simulink model "Inverter2Motor"  (R2025a)
settings: Solver=VariableStepAuto  StartTime=0.0  StopTime=5  RelTol=1e-3
model workspace (MAT data in the model file):
  CT_AmpersPerLSB = 0.0515718
  InverterVdc = 440
  Max_ADC_CNT = 4096
  MotorBaseCurrent = 20
  MotorKe = 0.031
  MotorLd = 0.000247
  MotorLq = 0.000371
  MotorPoles = 4
  MotorRs = 0.126
  PI_params_idKi = 1000
  PI_params_idKp = 0.4
  PI_params_iqKi = 1000
  PI_params_iqKp = 0.6
  Ts = 5e-05
libraries: simulink x3, slpidlib x2, mcbplantlib x1, autolibpmsminterior x1, mcbcontrolslib x1, dspstat3 x1, mcbcontrollergainlib x1, spsRMSLib x1, mcbeeMathTransformLib x1
settings Model: Creator=taiji  LastModifiedBy=taiji
settings DebuggingCC: ParamSuppressDoubleToSinglePrecisionLossMsg=on
settings RTWCC: GenCodeOnly=on  Toolchain=MinGW64 | gmake (64-bit Windows)

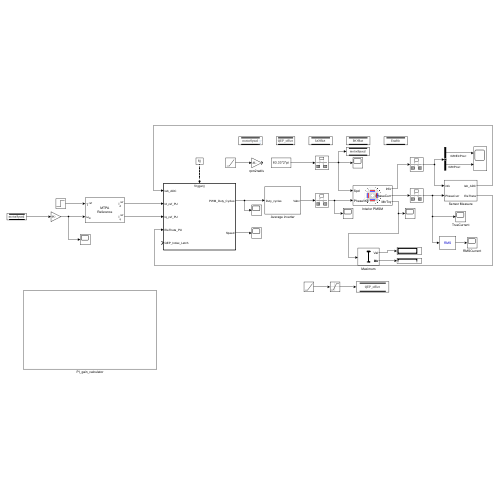
[thumbnail: Simulink's stored preview of the top-level diagram]
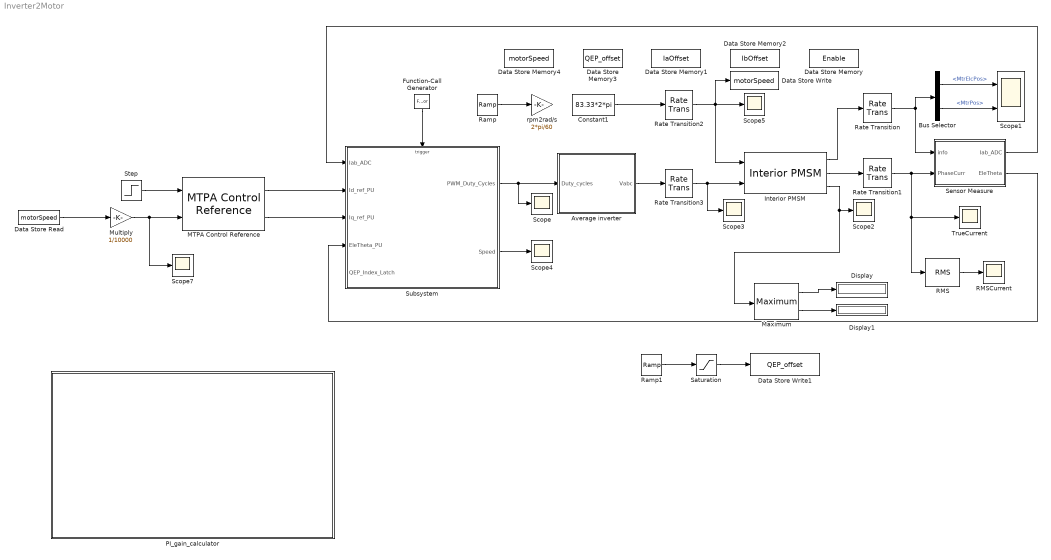
== system Inverter2Motor ==
  Average inverter : Subsystem
  Bus Selector : BusSelector  OutputSignals=MtrElcPos,MtrPos
  Constant1 : Constant  Value=83.33*2*pi
  Data Store Memory : DataStoreMemory  DataStoreName=Enable  WriteAfterWriteMsg=warning  InitialValue=1  ShowAdditionalParam=off  OutDataTypeStr=boolean
  Data Store Memory1 : DataStoreMemory  DataStoreName=IaOffset  WriteAfterWriteMsg=warning  ShowAdditionalParam=off  OutDataTypeStr=boolean
  Data Store Memory2 : DataStoreMemory  DataStoreName=IbOffset  WriteAfterWriteMsg=warning  ShowAdditionalParam=off  OutDataTypeStr=boolean
  Data Store Memory3 : DataStoreMemory  DataStoreName=QEP_offset  WriteAfterWriteMsg=warning  ShowAdditionalParam=off
  Data Store Memory4 : DataStoreMemory  DataStoreName=motorSpeed  WriteAfterWriteMsg=warning  ShowAdditionalParam=off
  Data Store Read : DataStoreRead  DataStoreName=motorSpeed  IndexOptions=Index vector (dialog)  Indices=1  OutputSizes=1
  Data Store Write : DataStoreWrite  DataStoreName=motorSpeed  IndexOptions=Index vector (dialog)  Indices=1  OutputSizes=1
  Data Store Write1 : DataStoreWrite  DataStoreName=QEP_offset  IndexOptions=Index vector (dialog)  Indices=1  OutputSizes=1
  Display : Display
  Display1 : Display
  Function-Call Generator : FunctionCallGenerator  SampleTime=Ts
  Interior PMSM : autolibpmsminterior/Interior PMSM  port_config=Speed  sim_type=Continuous  Ts=Ts  P=MotorPoles  Rs=MotorRs  Ldq=[MotorLd MotorLq]  KConstText=Back-emf constant (Ke):  lambda_pm=0.0427  Ke=MotorKe*1000*1.414  mechanical=[0.33e-3,4.924e-4,0]  idq0=[0 0]  theta_init=0  omega_init=0  KConst=MotorKe  lambda_pm_calc=0.060417  Kt=0.07  RefBlkName='autolibpmsminterior/Interior PMSM'  aMode=5
      settings: LibrarySourceBlock=mcblib/Electrical Systems/Motors/Interior PMSM
  MTPA Control Reference : mcbcontrolslib/MTPA Control Reference  VariantSelect=Interior PMSM  polePairs=MotorPoles  Rs=MotorRs  Ld=MotorLd  Lq=MotorLq  FluxPM=4.22e-2  ilimit=MotorBaseCurrent  Vdc_input_select=Specify via dialog  V_dc=InverterVdc  Units=Per-Unit (PU)  N_base=10000  I_base=MotorBaseCurrent  T_base=5.064  V_base=InverterVdc  N_base_disp=3182  MTPAiterator=on  iterCount=10
      settings: LibrarySourceBlock=mcblib/Controls/Control Reference/MTPA Control Reference
  Maximum : dspstat3/Maximum  operation=maximum  fcn=Value and Index  indexBase=Zero  operateOver=Entire input  Dimension=1  InputProcessing=Columns as channels (frame based)  reset=None  roiEnable=off  roiType=Rectangles  roiPortion=Entire ROI  roiOutput=Individual statistics for each ROI  roiFlag=off  roundingMode=Floor  overflowMode=off  accumDataTypeStr=Inherit: Same as product output  accumLastDataTypeStr=Inherit: Same as product output
      settings: LibrarySourceBlock=dsphdlsupportstat/Maximum
  Multiply : Gain  Gain=1/10000
  PI_gain_calculator : Subsystem
  RMS : spsRMSLib/RMS  TrueRMS=on  Freq=10  RMSInit=1  Ts=0
  RMSCurrent : Scope
      settings: ActiveDisplayYMinimum=-4.25669  ActiveDisplayYMaximum=48.31018
  Ramp : simulink/Sources/Ramp  slope=100  start=0  InitialOutput=0
  Ramp1 : simulink/Sources/Ramp  slope=0.2  start=0  InitialOutput=0
  Rate Transition{,1..3} (4 alike) : RateTransition
  Saturation : Saturate  UpperLimit=1  LowerLimit=0
  Scope{,2..5,7} (6 alike) : Scope
      Scope settings: ActiveDisplayYMinimum=0.31894  ActiveDisplayYMaximum=0.68106
      Scope2 settings: ActiveDisplayYMinimum=-45.02589  ActiveDisplayYMaximum=34.78623  DataLoggingVariableName=ScopeData2
      Scope3 settings: ActiveDisplayYMinimum=-8.9708136310234838  ActiveDisplayYMaximum=15.396875475913742  DataLoggingVariableName=ScopeData3
      Scope4 settings: ActiveDisplayYMinimum=-1  ActiveDisplayYMaximum=1  DataLoggingVariableName=ScopeData2
      Scope5 settings: ActiveDisplayYMinimum=0.0531  ActiveDisplayYMaximum=20.0531  DataLoggingVariableName=ScopeData9
      Scope7 settings: ActiveDisplayYMinimum=-1  ActiveDisplayYMaximum=1  DataLoggingVariableName=ScopeData2
  Scope1 : Scope  NumInputPorts=2
      settings: ActiveDisplayYMinimum=-0.25123  ActiveDisplayYMaximum=2.26104
  Sensor Measure : Subsystem
  Step : Step  SampleTime=0
  Subsystem : Subsystem
  TrueCurrent : Scope
      settings: ActiveDisplayYMinimum=-18.31363960222458  ActiveDisplayYMaximum=27.186348713788568  DataLoggingVariableName=ScopeData7
  rpm2rad/s : Gain  Gain=2*pi/60
  wires:
  Interior PMSM/1 -> Rate Transition/1
  Interior PMSM/2 -> Rate Transition1/1
  Average inverter/1(Vabc) -> Rate Transition3/1
  Rate Transition/1 -> Bus Selector/1, Sensor Measure/1(info)
  Rate Transition1/1 -> RMS/1, TrueCurrent/1, Sensor Measure/2(PhaseCurr)
  Sensor Measure/1(Iab_ADC) -> Subsystem/1(Iab_ADC)
  Bus Selector/1 -> Scope1/1  "<MtrElcPos>"
  Rate Transition3/1 -> Interior PMSM/2, Scope3/1
  Function-Call Generator/1 -> Subsystem/Trigger
  Subsystem/1(PWM_Duty_Cycles) -> Scope/1, Average inverter/1(Duty_cycles)
  Sensor Measure/2(EleTheta) -> Subsystem/4(EleTheta_PU)
  Interior PMSM/3 -> Maximum/1, Scope2/1
  RMS/1 -> RMSCurrent/1
  Subsystem/2(Speed) -> Scope4/1
  Step/1 -> MTPA Control Reference/1
  Ramp/1 -> rpm2rad/s/1
  MTPA Control Reference/1 -> Subsystem/2(Id_ref_PU)
  MTPA Control Reference/2 -> Subsystem/3(Iq_ref_PU)
  Rate Transition2/1 -> Interior PMSM/1, Data Store Write/1, Scope5/1
  Multiply/1 -> Scope7/1, MTPA Control Reference/2
  Data Store Read/1 -> Multiply/1
  Constant1/1 -> Rate Transition2/1
  Bus Selector/2 -> Scope1/2  "<MtrPos>"
  Ramp1/1 -> Saturation/1
  Saturation/1 -> Data Store Write1/1
  Maximum/1 -> Display/1
  Maximum/2 -> Display1/1

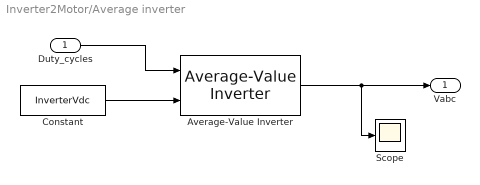
== system Inverter2Motor/Average inverter ==
  Duty_cycles : Inport
  Average-Value Inverter : mcbplantlib/Average-Value Inverter
      settings: LibrarySourceBlock=mcblib/Electrical Systems/Inverters/Average-Value Inverter
  Constant : Constant  Value=InverterVdc
  Scope : Scope
      settings: ActiveDisplayYMinimum=-91.90703  ActiveDisplayYMaximum=87.39239  DataLoggingVariableName=ScopeData6
  Vabc : Outport
  wires:
  Duty_cycles/1 -> Average-Value Inverter/1
  Constant/1 -> Average-Value Inverter/2
  Average-Value Inverter/1 -> Scope/1, Vabc/1

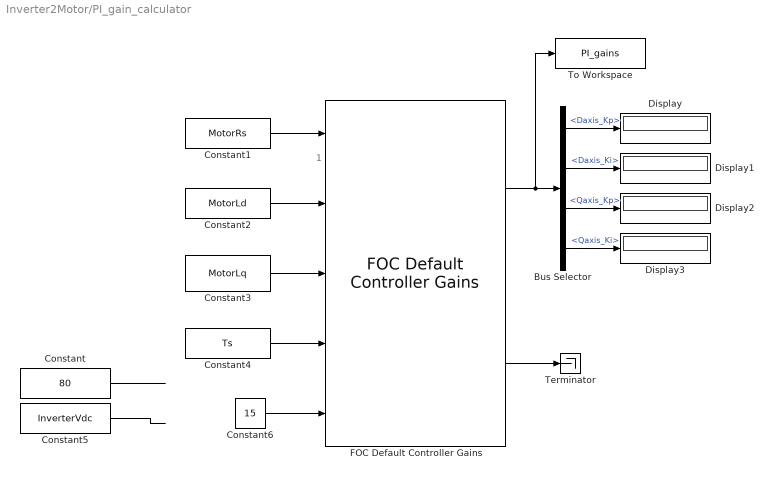
== system Inverter2Motor/PI_gain_calculator ==
  note: 1
  Bus Selector : BusSelector  OutputSignals=Daxis_Kp,Daxis_Ki,Qaxis_Kp,Qaxis_Ki
  Constant : Constant  Value=80
  Constant1 : Constant  Value=MotorRs
  Constant2 : Constant  Value=MotorLd
  Constant3 : Constant  Value=MotorLq
  Constant4 : Constant  Value=Ts  VectorParams1D=off
  Constant5 : Constant  Value=InverterVdc
  Constant6 : Constant  Value=15
  Display{,1..3} (4 alike) : Display
  FOC Default Controller Gains : mcbcontrollergainlib/FOC Default Controller Gains  ControllerGainType=Empirical method  motorSelection=PMSM  unitType=SI Unit  outCurrentControlGain=on  outFWCGain=off  outSpeedControlGain=off  externalDelay=off  currentSensorDelay=50e-6  speedSensorDelay=50e-6  speedFilterDelay=0.02
      settings: LibrarySourceBlock=mcblib/Controls/Controllers/FOC Default Controller Gains
  Terminator : Terminator
  To Workspace : ToWorkspace  VariableName=PI_gains  SaveFormat=Structure  SampleTime=-1
      settings: Save2DSignal=2-D array (concatenate along first dimension)
  wires:
  FOC Default Controller Gains/1 -> To Workspace/1, Bus Selector/1
  FOC Default Controller Gains/2 -> Terminator/1
  Constant6/1 -> FOC Default Controller Gains/5
  Constant4/1 -> FOC Default Controller Gains/4
  Constant3/1 -> FOC Default Controller Gains/3
  Constant2/1 -> FOC Default Controller Gains/2
  Constant1/1 -> FOC Default Controller Gains/1
  Constant/1 -> ?
  Constant5/1 -> ?
  Bus Selector/1 -> Display/1  "<Daxis_Kp>"
  Bus Selector/2 -> Display1/1  "<Daxis_Ki>"
  Bus Selector/3 -> Display2/1  "<Qaxis_Kp>"
  Bus Selector/4 -> Display3/1  "<Qaxis_Ki>"

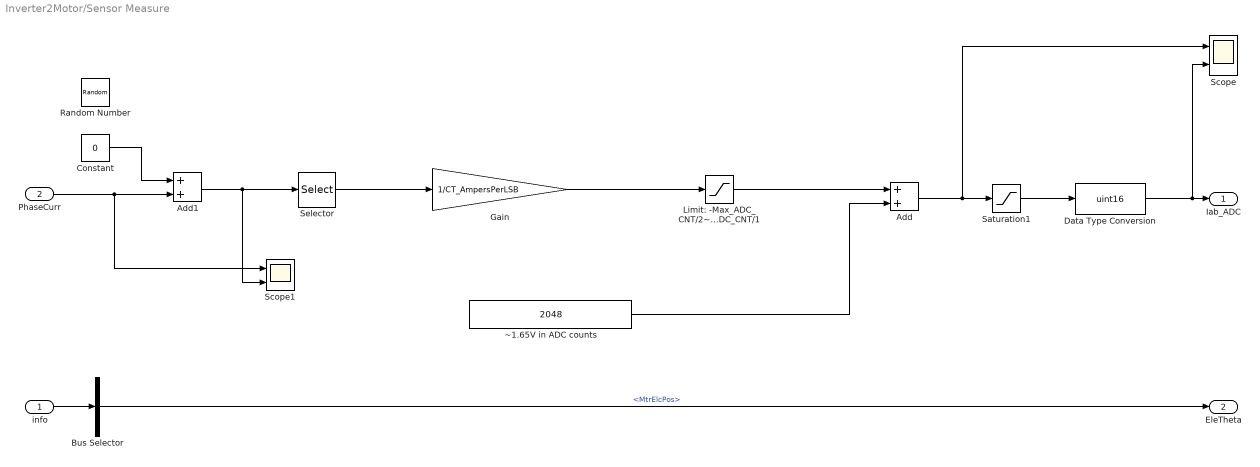
== system Inverter2Motor/Sensor Measure ==
  info : Inport
  PhaseCurr : Inport  Port=2
  Add : Sum
  Add1 : Sum
  Bus Selector : BusSelector  OutputSignals=MtrElcPos
  Constant : Constant  Value=0
  Data Type Conversion : DataTypeConversion  OutDataTypeStr=uint16  SaturateOnIntegerOverflow=off  RndMeth=Floor
  Gain : Gain  Gain=1/CT_AmpersPerLSB
  Limit: -Max_ADC_CNT/2~Max_ADC_CNT/1 : Saturate  UpperLimit=Max_ADC_CNT/2  LowerLimit=-Max_ADC_CNT/2
  Random Number : RandomNumber  Variance=0.1  SampleTime=0.00002
  Saturation1 : Saturate  UpperLimit=Max_ADC_CNT  LowerLimit=0
  Scope : Scope  NumInputPorts=2
      settings: ActiveDisplayYMinimum=-482.69811  ActiveDisplayYMaximum=3705.31296
  Scope1 : Scope  NumInputPorts=2
      settings: ActiveDisplayYMinimum=45.76188  ActiveDisplayYMaximum=65.93706
  Selector : Selector  InputPortWidth=3  IndexOptions=Index vector (dialog)  Indices=[1 2]  OutputSizes=1  RuntimeRangeChecks=on
  ~1.65V in ADC counts : Constant  Value=2048
  Iab_ADC : Outport
  EleTheta : Outport  Port=2
  wires:
  Gain/1 -> Limit: -Max_ADC_CNT/2~Max_ADC_CNT/1/1
  Saturation1/1 -> Data Type Conversion/1
  Add/1 -> Scope/1, Saturation1/1
  Limit: -Max_ADC_CNT/2~Max_ADC_CNT/1/1 -> Add/1
  ~1.65V in ADC counts/1 -> Add/2
  Selector/1 -> Gain/1
  Data Type Conversion/1 -> Scope/2, Iab_ADC/1
  info/1 -> Bus Selector/1
  Bus Selector/1 -> EleTheta/1  "<MtrElcPos>"
  PhaseCurr/1 -> Scope1/1, Add1/2
  Add1/1 -> Scope1/2, Selector/1
  Constant/1 -> Add1/1

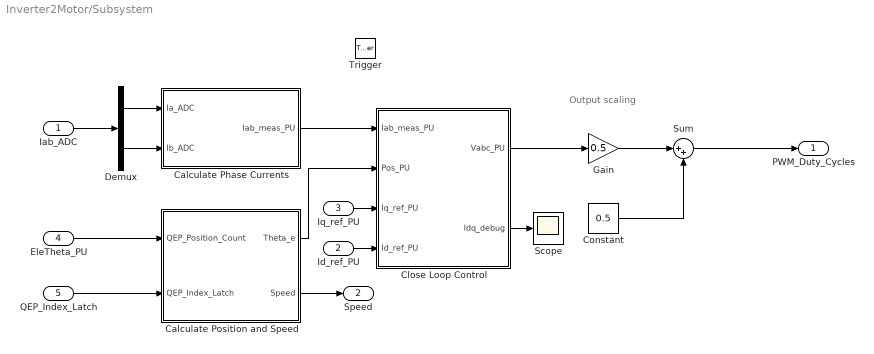
== system Inverter2Motor/Subsystem ==
  note: Output scaling
  Iab_ADC : Inport
  Id_ref_PU : Inport  Port=2
  Iq_ref_PU : Inport  Port=3
  EleTheta_PU : Inport  Port=4
  QEP_Index_Latch : Inport  Port=5
  Trigger : TriggerPort  TriggerType=function-call  VariantControl=(inherit)  PortDimensions=1
  Calculate Phase Currents : Subsystem
  Calculate Position and Speed : Subsystem
  Close Loop Control : Subsystem
  Constant : Constant  Value=0.5
  Demux : Demux  Outputs=2
  Gain : Gain  Gain=0.5
  Scope : Scope
      settings: ActiveDisplayYMinimum=-12.55833  ActiveDisplayYMaximum=58.23895  DataLoggingVariableName=ScopeData8
  Sum : Sum  Inputs=|++
  PWM_Duty_Cycles : Outport
  Speed : Outport  Port=2
  wires:
  Demux/2 -> Calculate Phase Currents/2(Ib_ADC)
  Calculate Position and Speed/1(Theta_e) -> Close Loop Control/2(Pos_PU)
  Demux/1 -> Calculate Phase Currents/1(Ia_ADC)
  Constant/1 -> Sum/2
  Calculate Phase Currents/1(Iab_meas_PU) -> Close Loop Control/1(Iab_meas_PU)
  Sum/1 -> PWM_Duty_Cycles/1
  Iab_ADC/1 -> Demux/1
  Close Loop Control/1(Vabc_PU) -> Gain/1
  Close Loop Control/2(Idq_debug) -> Scope/1
  Calculate Position and Speed/2(Speed) -> Speed/1
  Gain/1 -> Sum/1
  EleTheta_PU/1 -> Calculate Position and Speed/1(QEP_Position_Count)
  QEP_Index_Latch/1 -> Calculate Position and Speed/2(QEP_Index_Latch)
  Iq_ref_PU/1 -> Close Loop Control/3(Iq_ref_PU)
  Id_ref_PU/1 -> Close Loop Control/4(Id_ref_PU)

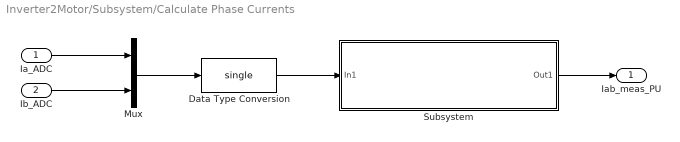
== system Inverter2Motor/Subsystem/Calculate Phase Currents ==
  Ia_ADC : Inport
  Ib_ADC : Inport  Port=2
  Data Type Conversion : DataTypeConversion  OutDataTypeStr=single  RndMeth=Floor
  Mux : Mux  Inputs=2
  Subsystem : Subsystem
  Iab_meas_PU : Outport
  wires:
  Ia_ADC/1 -> Mux/1
  Ib_ADC/1 -> Mux/2
  Mux/1 -> Data Type Conversion/1
  Subsystem/1(Out1) -> Iab_meas_PU/1
  Data Type Conversion/1 -> Subsystem/1(In1)

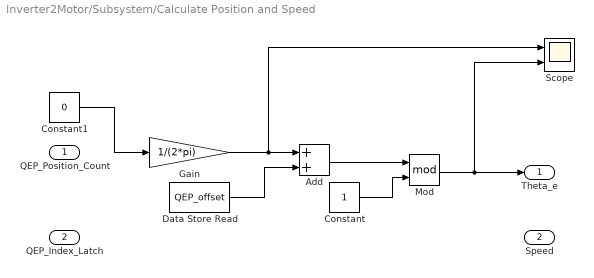
== system Inverter2Motor/Subsystem/Calculate Position and Speed ==
  QEP_Position_Count : Inport
  QEP_Index_Latch : Inport  Port=2
  Add : Sum
  Constant : Constant
  Constant1 : Constant  Value=0
  Data Store Read : DataStoreRead  DataStoreName=QEP_offset  IndexOptions=Index vector (dialog)  Indices=1  OutputSizes=1
  Gain : Gain  Gain=1/(2*pi)  OutDataTypeStr=Inherit: Same as input
  Mod : Math  Operator=mod
  Scope : Scope  NumInputPorts=2
      settings: ActiveDisplayYMinimum=-1  ActiveDisplayYMaximum=1
  Theta_e : Outport
  Speed : Outport  Port=2
  wires:
  Gain/1 -> Scope/1, Add/1
  Constant/1 -> Mod/2
  Add/1 -> Mod/1
  Data Store Read/1 -> Add/2
  Mod/1 -> Theta_e/1, Scope/2
  Constant1/1 -> Gain/1

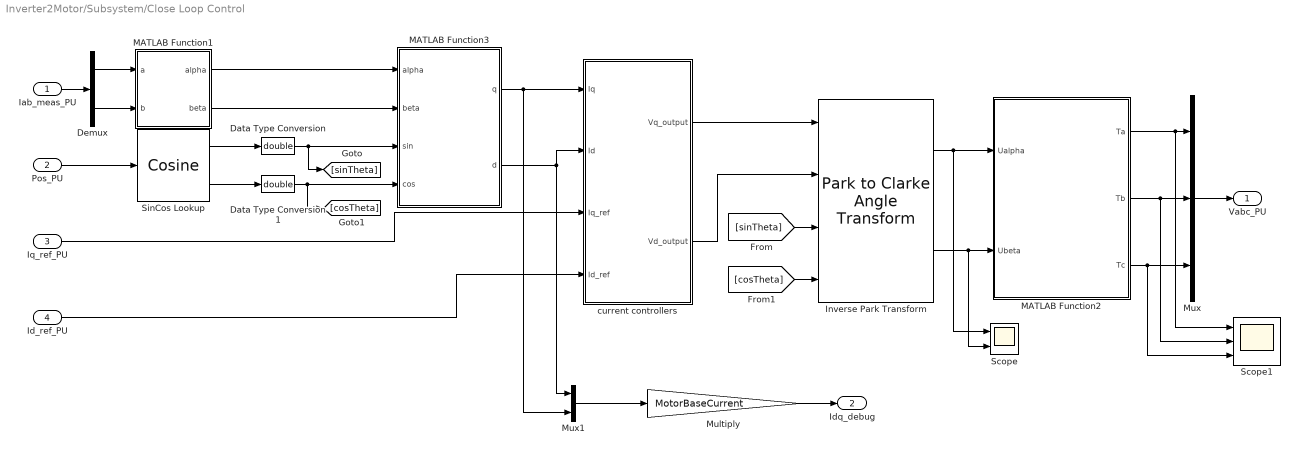
== system Inverter2Motor/Subsystem/Close Loop Control ==
  Iab_meas_PU : Inport
  Pos_PU : Inport  Port=2
  Iq_ref_PU : Inport  Port=3
  Id_ref_PU : Inport  Port=4
  Data Type Conversion : DataTypeConversion  OutDataTypeStr=double  SaturateOnIntegerOverflow=off  RndMeth=Floor
  Data Type Conversion1 : DataTypeConversion  OutDataTypeStr=double  SaturateOnIntegerOverflow=off  RndMeth=Floor
  Demux : Demux  Outputs=2
  Inverse Park Transform : mcbeeMathTransformLib/Park to Clarke Angle Transform  AxisAlignment=D-axis  UseWithEmbedded=on  PhaseInput=Two inputs  ThetaInput=Sine and Cosine electrical position  AngleInput=Per-unit  N_points=1024
      settings: LibrarySourceBlock=mcbcontrolslib/Inverse Park Transform
  MATLAB Function1 : MATLAB Function  TreatAsAtomicUnit=on
  MATLAB Function2 : MATLAB Function  TreatAsAtomicUnit=on
  MATLAB Function3 : MATLAB Function  TreatAsAtomicUnit=on
  Multiply : Gain  Gain=MotorBaseCurrent
  Mux : Mux  Inputs=3
  Mux1 : Mux  Inputs=2
  Scope : Scope  NumInputPorts=2
      settings: ActiveDisplayYMinimum=-0.06117  ActiveDisplayYMaximum=0.3667  DataLoggingVariableName=ScopeData11
  Scope1 : Scope  NumInputPorts=3
      settings: ActiveDisplayYMinimum=-0.03923  ActiveDisplayYMaximum=0.03927
  SinCos Lookup : simulink/Lookup Tables/Cosine  Formula=sin(2*pi*u) and cos(2*pi*u)  NumDataPoints=(2^5)+1  OutputWordLength=16  InternalRulePriority=Speed
      settings: LibrarySourceBlock=|
      | simulink/Quick Insert/Lookup
      | Tables/SinCos Lookup
  current controllers : Subsystem
  Vabc_PU : Outport
  Idq_debug : Outport  Port=2
  wires:
  SinCos Lookup/1 -> Data Type Conversion/1
  SinCos Lookup/2 -> Data Type Conversion1/1
  MATLAB Function3/1(q) -> current controllers/1(Iq), Mux1/2
  MATLAB Function1/1(alpha) -> MATLAB Function3/1(alpha)
  MATLAB Function1/2(beta) -> MATLAB Function3/2(beta)
  current controllers/1(Vq_output) -> Inverse Park Transform/1
  current controllers/2(Vd_output) -> Inverse Park Transform/2
  [cosTheta] -> Inverse Park Transform/4
  [sinTheta] -> Inverse Park Transform/3
  Inverse Park Transform/2 -> MATLAB Function2/2(Ubeta), Scope/2
  Iab_meas_PU/1 -> Demux/1
  Demux/2 -> MATLAB Function1/2(b)
  Demux/1 -> MATLAB Function1/1(a)
  Pos_PU/1 -> SinCos Lookup/1
  Iq_ref_PU/1 -> current controllers/3(Iq_ref)
  Mux/1 -> Vabc_PU/1
  MATLAB Function3/2(d) -> current controllers/2(Id), Mux1/1
  Mux1/1 -> Multiply/1
  Inverse Park Transform/1 -> MATLAB Function2/1(Ualpha), Scope/1
  Id_ref_PU/1 -> current controllers/4(Id_ref)
  Multiply/1 -> Idq_debug/1
  MATLAB Function2/1(Ta) -> Mux/1, Scope1/1
  MATLAB Function2/2(Tb) -> Mux/2, Scope1/2
  MATLAB Function2/3(Tc) -> Mux/3, Scope1/3
  Data Type Conversion/1 -> MATLAB Function3/3(sin), [sinTheta]
  Data Type Conversion1/1 -> MATLAB Function3/4(cos), [cosTheta]

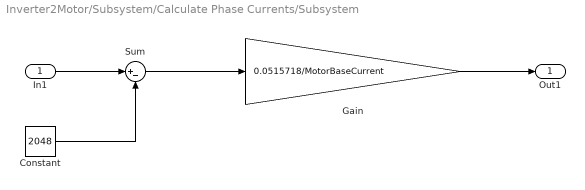
== system Inverter2Motor/Subsystem/Calculate Phase Currents/Subsystem ==
  In1 : Inport
  Constant : Constant  Value=2048
  Gain : Gain  Gain=0.0515718/MotorBaseCurrent  OutDataTypeStr=Inherit: Same as input
  Sum : Sum  Inputs=|+-
  Out1 : Outport
  wires:
  In1/1 -> Sum/1
  Gain/1 -> Out1/1
  Sum/1 -> Gain/1
  Constant/1 -> Sum/2

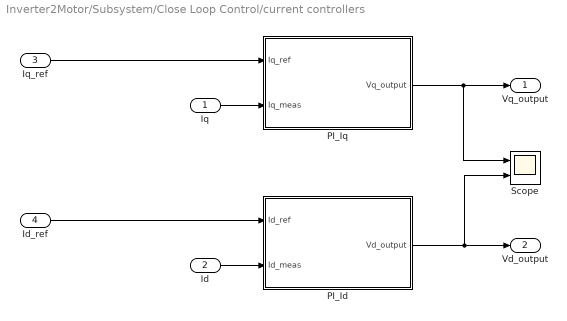
== system Inverter2Motor/Subsystem/Close Loop Control/current controllers ==
  Iq : Inport
  Id : Inport  Port=2
  Iq_ref : Inport  Port=3
  Id_ref : Inport  Port=4
  PI_Id : Subsystem
  PI_Iq : Subsystem
  Scope : Scope  NumInputPorts=2
      settings: ActiveDisplayYMinimum=-0.093  ActiveDisplayYMaximum=0.837  DataLoggingVariableName=ScopeData12
  Vq_output : Outport
  Vd_output : Outport  Port=2
  wires:
  PI_Iq/1(Vq_output) -> Scope/1, Vq_output/1
  PI_Id/1(Vd_output) -> Scope/2, Vd_output/1
  Id/1 -> PI_Id/2(Id_meas)
  Iq/1 -> PI_Iq/2(Iq_meas)
  Iq_ref/1 -> PI_Iq/1(Iq_ref)
  Id_ref/1 -> PI_Id/1(Id_ref)

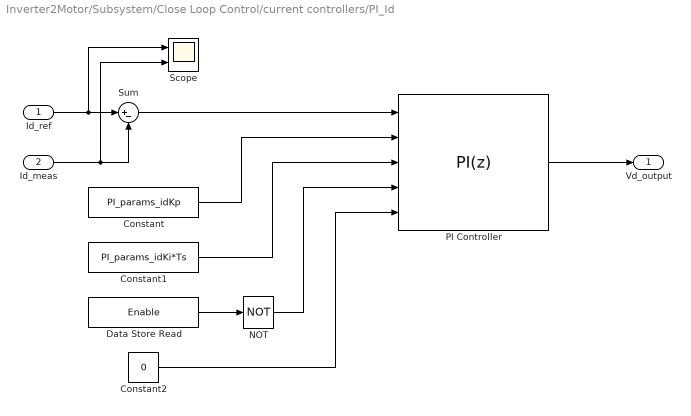
== system Inverter2Motor/Subsystem/Close Loop Control/current controllers/PI_Id ==
  Id_ref : Inport
  Id_meas : Inport  Port=2
  Constant : Constant  Value=PI_params_idKp
  Constant1 : Constant  Value=PI_params_idKi*Ts
  Constant2 : Constant  Value=0
  Data Store Read : DataStoreRead  DataStoreName=Enable  IndexOptions=Index vector (dialog)  Indices=1  OutputSizes=1
  NOT : Logic  Operator=NOT  IconShape=distinctive  AllPortsSameDT=off  OutDataTypeStr=boolean
  PI Controller : slpidlib/PID Controller  Controller=PI  Form=Parallel  TimeDomain=Discrete-time  UseExternalTs=off  SampleTime=-1  IntegratorMethod=Forward Euler  FilterMethod=Forward Euler  ControllerParametersSource=external  P=1  I=1  UseKiTs=on  D=0  UseExternalDerivativeSource=off  N=100  UseFilter=on  TunerSelectOption=Transfer Function Based (PID Tuner App)  InitialConditionSource=external  InitialConditionForIntegrator=0  InitialConditionForFilter=0  DifferentiatorICPrevScaledInput=0  ExternalReset=level  TrackingMode=off  Kt=1  LimitOutput=on  SatLimitsSource=internal  UpperSaturationLimit=1  LowerSaturationLimit=-1  LinearizeAsGain=on  AntiWindupMode=clamping  Kb=1  LimitIntegrator=on  UpperIntegratorSaturationLimit=1  LowerIntegratorSaturationLimit=-1  RndMeth=Simplest  POutMin=[]  POutMax=[]  IOutMin=[]  IOutMax=[]  DOutMin=[]  DOutMax=[]  NOutMin=[]  NOutMax=[]  SumOutMin=[]  SumOutMax=[]  SaturationOutDataTypeStr=Inherit: Inherit via back propagation  SaturationOutMin=[]  SaturationOutMax=[]  PParamMin=[]  PParamMax=[]  IParamMin=[]  IParamMax=[]  DParamMin=[]  DParamMax=[]  NParamMin=[]  NParamMax=[]  KbParamMin=[]  KbParamMax=[]  KtParamMin=[]  KtParamMax=[]  KbOutMin=[]  KbOutMax=[]  KtOutMin=[]  KtOutMax=[]  IntegratorOutMin=[]  IntegratorOutMax=[]  FilterOutMin=[]  FilterOutMax=[]  SumI1OutMin=[]  SumI1OutMax=[]  SumI2OutMin=[]  SumI2OutMax=[]  SumI3OutMin=[]  SumI3OutMax=[]  SumI4OutMin=[]  SumI4OutMax=[]  SumDOutMin=[]  SumDOutMax=[]  DifferentiatorOutMin=[]  DifferentiatorOutMax=[]  FilterDiffOutCoefMin=[]  FilterDiffOutCoefMax=[]  ReciprocalOutMin=[]  ReciprocalOutMax=[]  SumDenOutMin=[]  SumDenOutMax=[]  SumNumOutMin=[]  SumNumOutMax=[]  DivideOutMin=[]  DivideOutMax=[]  UdiffTsProdOutMin=[]  UdiffTsProdOutMax=[]  NTsProdOutMin=[]  NTsProdOutMax=[]  UintegralTsProdOutMin=[]  UintegralTsProdOutMax=[]  UngainTsProdOutMin=[]  UngainTsProdOutMax=[]  ClampingZeroOutDataTypeStr=Inherit: Inherit via back propagation  ClampingZeroOutMin=[]  ClampingZeroOutMax=[]  FilterDenConstantOutDataTypeStr=Inherit: Inherit via back propagation  FilterDenConstantOutMin=[]  FilterDenConstantOutMax=[]  PCopyOutDataTypeStr=Inherit: Inherit via back propagation  PCopyOutMin=[]  PCopyOutMax=[]  NCopyOutDataTypeStr=Inherit: Inherit via back propagation  NCopyOutMin=[]  NCopyOutMax=[]  IntegratorContinuousStateAttributes=''  IntegratorStateMustResolveToSignalObject=off  IntegratorRTWStateStorageClass=Auto  FilterContinuousStateAttributes=''  FilterStateMustResolveToSignalObject=off  FilterRTWStateStorageClass=Auto  ParallelPVariant=ExternalParameters  IdealPVariant=Disabled  IVariant=ExternalParameters  DVariant=Disabled  IntegratorVariant=Discrete  SatVariant=Enabled  AWVariant=DiscClampingParallel  PCopyVariant=Disabled  TRVariant=Disabled  FdbkBlocksVariant=Forward  IdealPFdbkVariant=Disabled  SatFdbkVariant=Disabled  DerivativeFilterVariant=Disabled  NVariant=Disabled  NCopyVariant=Disabled_SignalSpec  FilterICVariant=Disabled  IntegratorICVariant=ExternalICs  ExternalResetVariant=ExternalReset  TRSumVariant=Passthrough  SumFdbkVariant=Disabled  SumVariant=Sum_PI  TsampFilterVariant=InternalTs  TsampNgainVariant=Passthrough  TsampIntegralVariant=Disabled_SignalSpec  ExternalSaturationOutDataTypeStr=Inherit: Same as second input  DerivativeSourceVariant=Disabled  PreIntVariant=InternalPreInt
  Scope : Scope  NumInputPorts=2
      settings: ActiveDisplayYMinimum=-3.8890997761969657  ActiveDisplayYMaximum=12.162758850679191  DataLoggingVariableName=ScopeData10
  Sum : Sum  Inputs=|+-
  Vd_output : Outport
  wires:
  Id_ref/1 -> Scope/1, Sum/1
  Constant2/1 -> PI Controller/5
  NOT/1 -> PI Controller/4
  Id_meas/1 -> Scope/2, Sum/2
  Constant1/1 -> PI Controller/3
  Constant/1 -> PI Controller/2
  PI Controller/1 -> Vd_output/1
  Data Store Read/1 -> NOT/1
  Sum/1 -> PI Controller/1

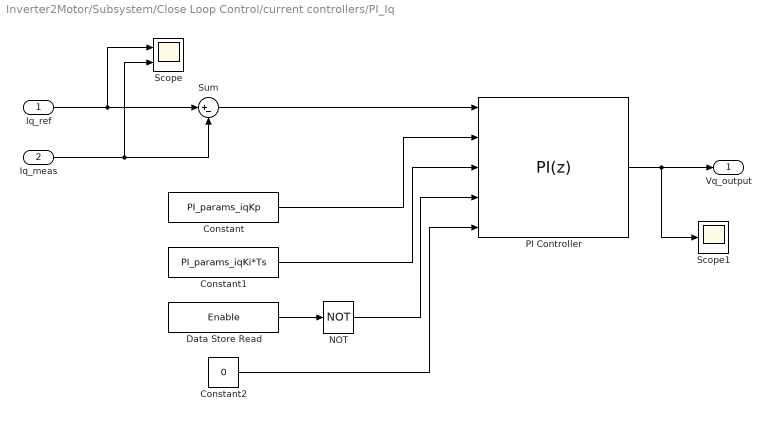
== system Inverter2Motor/Subsystem/Close Loop Control/current controllers/PI_Iq ==
  Iq_ref : Inport
  Iq_meas : Inport  Port=2
  Constant : Constant  Value=PI_params_iqKp
  Constant1 : Constant  Value=PI_params_iqKi*Ts
  Constant2 : Constant  Value=0
  Data Store Read : DataStoreRead  DataStoreName=Enable  IndexOptions=Index vector (dialog)  Indices=1  OutputSizes=1
  NOT : Logic  Operator=NOT  IconShape=distinctive  AllPortsSameDT=off  OutDataTypeStr=boolean
  PI Controller : slpidlib/PID Controller  Controller=PI  Form=Parallel  TimeDomain=Discrete-time  UseExternalTs=off  SampleTime=-1  IntegratorMethod=Forward Euler  FilterMethod=Forward Euler  ControllerParametersSource=external  P=1  I=1  UseKiTs=on  D=0  UseExternalDerivativeSource=off  N=100  UseFilter=on  TunerSelectOption=Transfer Function Based (PID Tuner App)  InitialConditionSource=external  InitialConditionForIntegrator=0  InitialConditionForFilter=0  DifferentiatorICPrevScaledInput=0  ExternalReset=level  TrackingMode=off  Kt=1  LimitOutput=on  SatLimitsSource=internal  UpperSaturationLimit=1  LowerSaturationLimit=-1  LinearizeAsGain=on  AntiWindupMode=clamping  Kb=1  LimitIntegrator=on  UpperIntegratorSaturationLimit=1  LowerIntegratorSaturationLimit=-1  RndMeth=Simplest  POutMin=[]  POutMax=[]  IOutMin=[]  IOutMax=[]  DOutMin=[]  DOutMax=[]  NOutMin=[]  NOutMax=[]  SumOutMin=[]  SumOutMax=[]  SaturationOutDataTypeStr=Inherit: Inherit via back propagation  SaturationOutMin=[]  SaturationOutMax=[]  PParamMin=[]  PParamMax=[]  IParamMin=[]  IParamMax=[]  DParamMin=[]  DParamMax=[]  NParamMin=[]  NParamMax=[]  KbParamMin=[]  KbParamMax=[]  KtParamMin=[]  KtParamMax=[]  KbOutMin=[]  KbOutMax=[]  KtOutMin=[]  KtOutMax=[]  IntegratorOutMin=[]  IntegratorOutMax=[]  FilterOutMin=[]  FilterOutMax=[]  SumI1OutMin=[]  SumI1OutMax=[]  SumI2OutMin=[]  SumI2OutMax=[]  SumI3OutMin=[]  SumI3OutMax=[]  SumI4OutMin=[]  SumI4OutMax=[]  SumDOutMin=[]  SumDOutMax=[]  DifferentiatorOutMin=[]  DifferentiatorOutMax=[]  FilterDiffOutCoefMin=[]  FilterDiffOutCoefMax=[]  ReciprocalOutMin=[]  ReciprocalOutMax=[]  SumDenOutMin=[]  SumDenOutMax=[]  SumNumOutMin=[]  SumNumOutMax=[]  DivideOutMin=[]  DivideOutMax=[]  UdiffTsProdOutMin=[]  UdiffTsProdOutMax=[]  NTsProdOutMin=[]  NTsProdOutMax=[]  UintegralTsProdOutMin=[]  UintegralTsProdOutMax=[]  UngainTsProdOutMin=[]  UngainTsProdOutMax=[]  ClampingZeroOutDataTypeStr=Inherit: Inherit via back propagation  ClampingZeroOutMin=[]  ClampingZeroOutMax=[]  FilterDenConstantOutDataTypeStr=Inherit: Inherit via back propagation  FilterDenConstantOutMin=[]  FilterDenConstantOutMax=[]  PCopyOutDataTypeStr=Inherit: Inherit via back propagation  PCopyOutMin=[]  PCopyOutMax=[]  NCopyOutDataTypeStr=Inherit: Inherit via back propagation  NCopyOutMin=[]  NCopyOutMax=[]  IntegratorContinuousStateAttributes=''  IntegratorStateMustResolveToSignalObject=off  IntegratorRTWStateStorageClass=Auto  FilterContinuousStateAttributes=''  FilterStateMustResolveToSignalObject=off  FilterRTWStateStorageClass=Auto  ParallelPVariant=ExternalParameters  IdealPVariant=Disabled  IVariant=ExternalParameters  DVariant=Disabled  IntegratorVariant=Discrete  SatVariant=Enabled  AWVariant=DiscClampingParallel  PCopyVariant=Disabled  TRVariant=Disabled  FdbkBlocksVariant=Forward  IdealPFdbkVariant=Disabled  SatFdbkVariant=Disabled  DerivativeFilterVariant=Disabled  NVariant=Disabled  NCopyVariant=Disabled_SignalSpec  FilterICVariant=Disabled  IntegratorICVariant=ExternalICs  ExternalResetVariant=ExternalReset  TRSumVariant=Passthrough  SumFdbkVariant=Disabled  SumVariant=Sum_PI  TsampFilterVariant=InternalTs  TsampNgainVariant=Passthrough  TsampIntegralVariant=Disabled_SignalSpec  ExternalSaturationOutDataTypeStr=Inherit: Same as second input  DerivativeSourceVariant=Disabled  PreIntVariant=InternalPreInt
      settings: LibrarySourceBlock=mcblib/Controls/Controllers/PI Controller
  Scope : Scope  NumInputPorts=2
      settings: ActiveDisplayYMinimum=-12.126194418834254  ActiveDisplayYMaximum=4.1136548322916493  DataLoggingVariableName=ScopeData4
  Scope1 : Scope
      settings: ActiveDisplayYMinimum=-0.0238  ActiveDisplayYMaximum=0.36485  DataLoggingVariableName=ScopeData5
  Sum : Sum  Inputs=|+-
  Vq_output : Outport
  wires:
  Iq_ref/1 -> Scope/1, Sum/1
  Constant2/1 -> PI Controller/5
  NOT/1 -> PI Controller/4
  Iq_meas/1 -> Scope/2, Sum/2
  Constant1/1 -> PI Controller/3
  Constant/1 -> PI Controller/2
  PI Controller/1 -> Scope1/1, Vq_output/1
  Data Store Read/1 -> NOT/1
  Sum/1 -> PI Controller/1

== matlab function Inverter2Motor/Subsystem/Close Loop Control/MATLAB Function1 ==
  data: a input; alpha output; beta output; b input
function [alpha, beta]= clarke(a, b)

alpha = a;
beta = (a+2*b)*0.57735026918963;

== matlab function Inverter2Motor/Subsystem/Close Loop Control/MATLAB Function3 ==
  data: q output; alpha input; d output; beta input; sin input; cos input
function [q, d]= park(alpha, beta, sin, cos)

d = alpha*cos + beta*sin;
q = beta*cos - alpha*sin;

== matlab function Inverter2Motor/Subsystem/Close Loop Control/MATLAB Function2 ==
  data: Ualpha input; Ubeta input; Ta output; Tb output; Tc output
function [Ta, Tb, Tc]= svgen(Ualpha, Ubeta)
    tmp1= Ubeta;															
    tmp2= Ubeta/2 + 0.866*Ualpha;					
    tmp3= tmp2 -  tmp1;												
															    
    VecSector = 3;
    if(tmp2> 0)
        VecSector = VecSector-1;
    end
    if (tmp3> 0)
        VecSector = VecSector-1;
    end
    if(tmp1< 0)
        VecSector = 7-VecSector;
    end

    if( VecSector==1 ||  VecSector==4)                                 
        Ta=  tmp2; 													
        Tb=  tmp1- tmp3; 												
        Tc=- tmp2;																		    								   																			
    elseif( VecSector==2 ||  VecSector==5)                                 
        Ta=  tmp3+ tmp2; 												
        Tb=  tmp1; 													
        Tc=- tmp1;																													   																			
    else                                                                    
        Ta=  tmp3; 													
        Tb=- tmp3; 													
        Tc=-( tmp1+ tmp2);												
    end
